simulink model "exam2_sim"  (R2023a)
settings: Solver=VariableStepAuto  StartTime=0.0  StopTime=10.0  RelTol=1e-3
undefined symbols (not defined in the file or in its folder): x10, x20
libraries: simulink x2
settings Model: Creator=laptop  LastModifiedBy=laptop

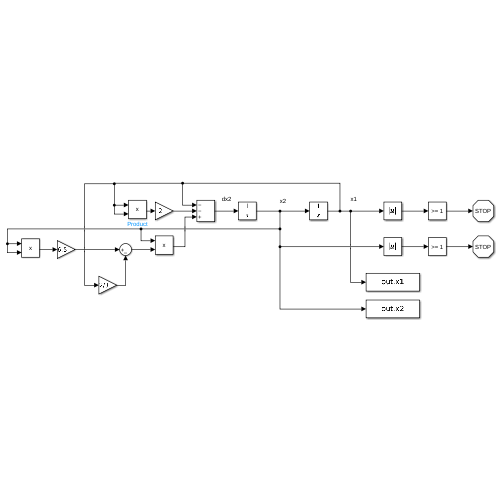
[thumbnail: Simulink's stored preview of the top-level diagram]
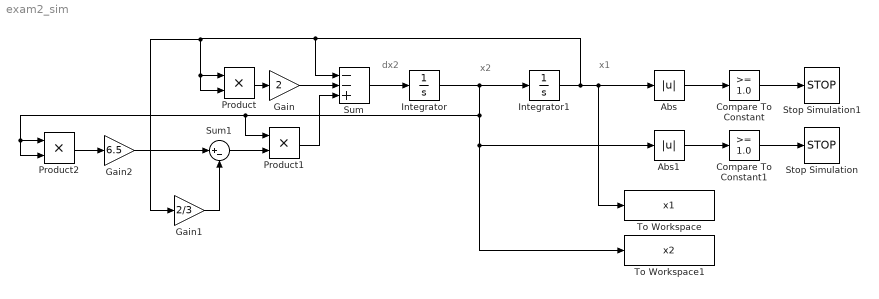
== system exam2_sim ==
  note: dx2
  note: x1
  note: x2
  Abs : Abs  SaturateOnIntegerOverflow=off
  Abs1 : Abs  SaturateOnIntegerOverflow=off
  Compare To Constant : simulink/Logic and Bit Operations/Compare To Constant  relop=>=  const=1.0  OutDataTypeStr=boolean
  Compare To Constant1 : simulink/Logic and Bit Operations/Compare To Constant  relop=>=  const=1.0  OutDataTypeStr=boolean
  Gain : Gain  Gain=2
  Gain1 : Gain  Gain=2/3
  Gain2 : Gain  Gain=6.5
  Integrator : Integrator  InitialCondition=x20
  Integrator1 : Integrator  InitialCondition=x10
  Product : Product
  Product1 : Product
  Product2 : Product
  Stop Simulation : Stop
  Stop Simulation1 : Stop
  Sum : Sum  Inputs=--+
  Sum1 : Sum  Inputs=|+-
  To Workspace : ToWorkspace  VariableName=x1  SampleTime=-1
  To Workspace1 : ToWorkspace  VariableName=x2  SampleTime=-1
  wires:
  Integrator/1 -> To Workspace1/1, Abs1/1, Product2/2, Product2/1, Product1/1, Integrator1/1
  Sum/1 -> Integrator/1
  Gain/1 -> Sum/2
  Product/1 -> Gain/1
  Integrator1/1 -> To Workspace/1, Abs/1, Sum/1, Gain1/1, Product/2, Product/1
  Product1/1 -> Sum/3
  Sum1/1 -> Product1/2
  Gain1/1 -> Sum1/2
  Gain2/1 -> Sum1/1
  Product2/1 -> Gain2/1
  Abs/1 -> Compare To Constant/1
  Abs1/1 -> Compare To Constant1/1
  Compare To Constant1/1 -> Stop Simulation/1
  Compare To Constant/1 -> Stop Simulation1/1
